simulink model "AM_Simulation"  (Simulink 6.5)
settings: Solver=ode45  StartTime=0.0  StopTime=1  RelTol=1e-3
undefined symbols (not defined in the file or in its folder): get
libraries: dspsrcs4 x5, simulink x2, dsparch4 x1, dspsnks4 x1
settings Model: Creator=shay  LastModifiedBy=jacobf

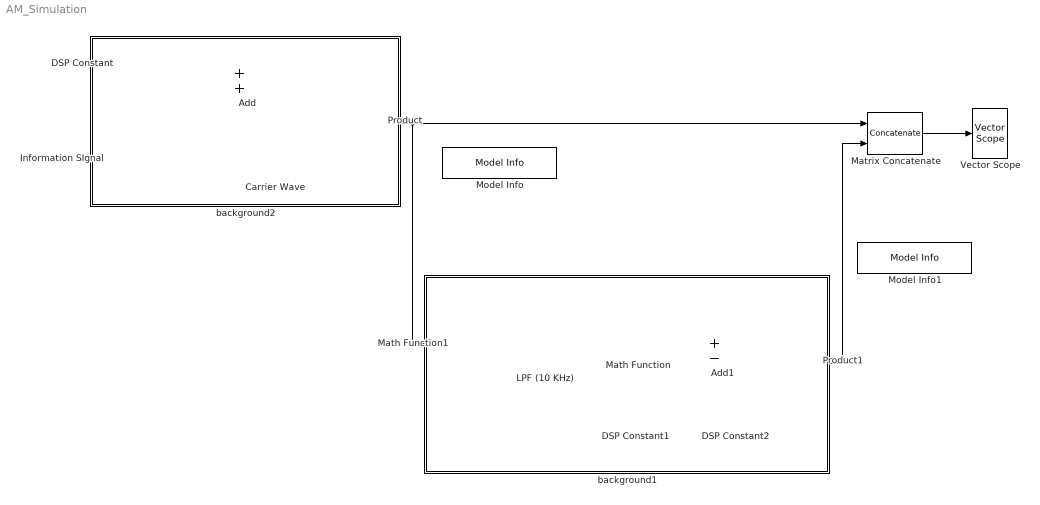
== system AM_Simulation ==
  Add : Sum  OutScaling=2^-10
  Add1 : Sum  Inputs=+-  OutScaling=2^-10
  Carrier Wave : dspsrcs4/Sine Wave  Amplitude=1  Frequency=15000  Phase=0  SampleMode=Discrete  OutComplex=Real  CompMethod=Trigonometric fcn  TableSize=Speed  SampleTime=1/96000  SamplesPerFrame=64  dataType=double  wordLen=16  udDataType=sfix(16)  fracBitsMode=Best precision  numFracBits=15  ResetState=Restart at time zero
  DSP Constant : dspsrcs4/DSP Constant  SystemSampleTime=-1  Value=1.5  SampleMode=Discrete  discreteOutput=Sample-based  continuousOutput=Sample-based  sampTime=1  framePeriod=2  dataType=Inherit from 'Constant value'  isSigned=on  wordLen=16  udDataType=sfix(16)  fracBitsMode=Best precision  numFracBits=15  InterpretAs1D=-inf  Ts=-inf  FramebasedOutput=-inf
  DSP Constant1 : dspsrcs4/DSP Constant  SystemSampleTime=-1  Value=1  SampleMode=Discrete  discreteOutput=Sample-based  continuousOutput=Sample-based  sampTime=1  framePeriod=2  dataType=Inherit from 'Constant value'  isSigned=on  wordLen=16  udDataType=sfix(16)  fracBitsMode=Best precision  numFracBits=15  InterpretAs1D=-inf  Ts=-inf  FramebasedOutput=-inf
  DSP Constant2 : dspsrcs4/DSP Constant  SystemSampleTime=-1  Value=2  SampleMode=Discrete  discreteOutput=Sample-based  continuousOutput=Sample-based  sampTime=1  framePeriod=2  dataType=Inherit from 'Constant value'  isSigned=on  wordLen=16  udDataType=sfix(16)  fracBitsMode=Best precision  numFracBits=15  InterpretAs1D=-inf  Ts=-inf  FramebasedOutput=-inf
  Information SIgnal : dspsrcs4/Sine Wave  Amplitude=1  Frequency=1000  Phase=0  SampleMode=Discrete  OutComplex=Real  CompMethod=Trigonometric fcn  TableSize=Speed  SampleTime=1/96000  SamplesPerFrame=64  dataType=double  wordLen=16  udDataType=sfix(16)  fracBitsMode=Best precision  numFracBits=15  ResetState=Restart at time zero
  LPF (10 KHz) : dsparch4/Digital Filter Design  SystemSampleTime=-1  mwdsp_browser_bugfix_var=off
  Math Function : Math  Operator=sqrt  SaturateOnIntegerOverflow=on
  Math Function1 : Math  Operator=square  SaturateOnIntegerOverflow=on
  Matrix Concatenate : Concatenate  Mode=Horizontal matrix concatenation
  Model Info : simulink/Model-Wide Utilities/Model Info  SystemSampleTime=-1  InitialBlockCM=None  BlockCM=None  Frame=on  DisplayStringWithTags=Modulated Signal  HorizontalTextAlignment=Center  LeftAlignmentValue=0.5  SourceBlockDiagram=AM_Simulation  TagMaxNumber=20
  Model Info1 : simulink/Model-Wide Utilities/Model Info  SystemSampleTime=-1  InitialBlockCM=None  BlockCM=None  Frame=on  DisplayStringWithTags=Demodulated Signal  HorizontalTextAlignment=Center  LeftAlignmentValue=0.5  SourceBlockDiagram=AM_Simulation  TagMaxNumber=20
  Product : Product  RndMeth=Zero
  Product1 : Product  RndMeth=Zero
  Vector Scope : dspsnks4/Vector Scope  DialogController=dspdialog.VectorScope  DialogControllerArgs=DataTag1  ScopeProperties=on  Domain=Time  HorizSpan=5  DisplayProperties=off  AxisGrid=on  Memory=off  FrameNumber=on  AxisLegend=off  AxisZoom=off  OpenScopeAtSimStart=on  OpenScopeImmediately=off  FigPos=get(0,'defaultfigureposition')  AxisProperties=off  XUnits=Hertz  XRange=[0...Fs/2]  InheritXIncr=on  XIncr=1  XLabel=Time  YUnits=dB  YLabel=Amplitude  LineProperties=off  LineDisables=on|on  LineColors=[0 0 1]|[1 0 0]
      settings: YMin=-2.62332794217152  YMax=2.55644562903253
  background1 : Subsystem
      settings: AttributesFormatString=AM Receiver
      mask Display: disp('')
  background2 : Subsystem
      settings: AttributesFormatString=AM Transmitter
      mask Display: disp('')
  wires:
  DSP Constant/1 -> Add/1
  Information SIgnal/1 -> Add/2
  Add/1 -> Product/1
  Carrier Wave/1 -> Product/2
  Product/1 -> Matrix Concatenate/1, Math Function1/1
  Matrix Concatenate/1 -> Vector Scope/1
  Product1/1 -> Matrix Concatenate/2
  DSP Constant2/1 -> Product1/2
  Add1/1 -> Product1/1
  Math Function/1 -> Add1/1
  DSP Constant1/1 -> Add1/2
  LPF (10 KHz)/1 -> Math Function/1
  Math Function1/1 -> LPF (10 KHz)/1

== system AM_Simulation/background1 ==

== system AM_Simulation/background2 ==
